simulink model "COBAN"  (R2018b)
settings: Solver=VariableStepAuto  StartTime=0.0  StopTime=15  RelTol=1e-3
model workspace (MAT data in the model file):
  K_1 = 100
  K_g = 0.1
  K_m = 2
  K_pot = 0.318
  a = 100
  a_m = 2
libraries: simulink x1
settings Model: OrderedModelArguments=off  Creator=alperdogan  LastModifiedBy=beyzanurcoban
settings SFSimCC: SimUseLocalCustomCode=off
settings RTWCC: RTWUseLocalCustomCode=off
settings CodeAppCC: StateflowObjectComments=on

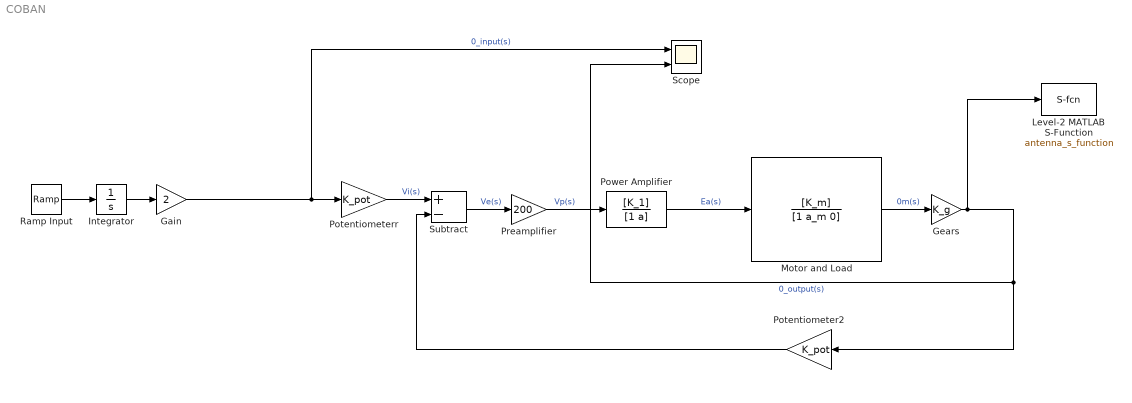
== system COBAN ==
  Gain : Gain  Gain=2
  Gears : Gain  Gain=K_g
  Integrator : Integrator
  Level-2 MATLAB S-Function : M-S-Function  FunctionName=antenna_s_function
  Motor and Load : TransferFcn  Numerator=[K_m]  Denominator=[1 a_m 0]
  Potentiometer2 : Gain  Gain=K_pot
  Potentiometerr : Gain  Gain=K_pot
  "Power Amplifier " : TransferFcn  Numerator=[K_1]  Denominator=[1 a]
  Preamplifier : Gain  Gain=200
  "Ramp Input " : simulink/Sources/Ramp  slope=1  start=0  InitialOutput=0
  Scope : Scope  NumInputPorts=2
  Subtract : Sum  Inputs=+-
  wires:
  "Power Amplifier "/1 -> Motor and Load/1  "Ea(s)"
  Motor and Load/1 -> Gears/1  "0m(s)"
  Preamplifier/1 -> "Power Amplifier "/1  "Vp(s)"
  Gears/1 -> Level-2 MATLAB S-Function/1, Scope/2, Potentiometer2/1  "0_output(s)"
  Potentiometer2/1 -> Subtract/2
  Subtract/1 -> Preamplifier/1  "Ve(s)"
  Potentiometerr/1 -> Subtract/1  "Vi(s)"
  "Ramp Input "/1 -> Integrator/1
  Integrator/1 -> Gain/1
  Gain/1 -> Scope/1, Potentiometerr/1  "0_input(s)"
